simulink model "fourteen_bus_dynamic"  (Simulink 7.8)
settings: Solver=ode23t  StartTime=0.0  StopTime=5  FixedStep=0.2  RelTol=1e-4  AbsTol=1e-6
undefined symbols (not defined in the file or in its folder): D1, Delta
libraries: powerlib x56
settings Model: Creator=Bharath  LastModifiedBy=Bharath
settings SolverCC: MaxConsecutiveMinStep=auto  ZeroCrossControl=DisableAll
settings DataIOCC: LimitDataPoints=off  MaxDataPoints=500000
settings DebuggingCC: SolverPrmCheckMsg=none  UnconnectedOutputMsg=none

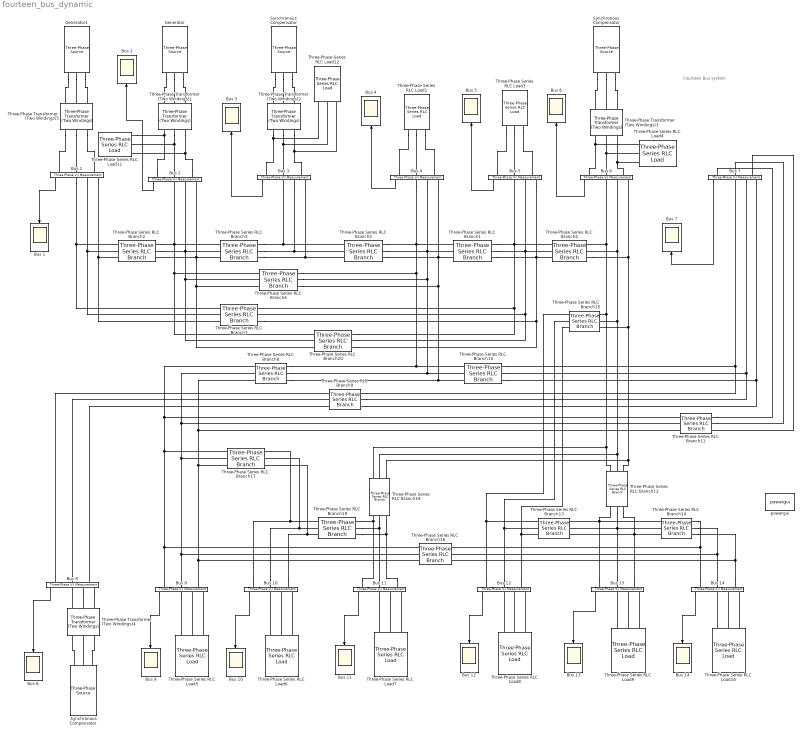
== system fourteen_bus_dynamic ==
  note: Fourteen Bus system
  " Generator" : powerlib/Electrical Sources/Three-Phase Source  Voltage=1.045  PhaseAngle=-30  Frequency=50  InternalConnection=Yg  SpecifyImpedance=on  Resistance=0.8929  Inductance=16.58e-3  ShortCircuitLevel=10  BaseVoltage=1  XRratio=1  BusType=PV  Pref=0.4  Qref=0  Qmin=-0.4  Qmax=0.5
  " Generator1" : powerlib/Electrical Sources/Three-Phase Source  Voltage=1.06  PhaseAngle=-30  Frequency=50  InternalConnection=Yg  SpecifyImpedance=on  Resistance=0.8929  Inductance=16.58e-3  ShortCircuitLevel=10  BaseVoltage=1  XRratio=1  BusType=PQ  Pref=2.324  Qref=-0.169  Qmin=0  Qmax=0
  Bus {1..14} (14 alike) : Scope
      Bus 1 settings: TimeRange=5  YMin=-1.75  YMax=1.75  SaveName=ScopeBus1
      Bus 10 settings: TimeRange=5  YMin=-1.5  YMax=1.5  SaveName=ScopeBus10
      Bus 11 settings: TickLabels=on  TimeRange=5  YMin=-1.25  YMax=1.25  SaveName=ScopeBus11
      Bus 12 settings: TimeRange=5  YMin=-1.25  YMax=1.25  SaveName=ScopeBus12
      Bus 13 settings: TimeRange=5  YMin=-1.25  YMax=1.25  SaveName=ScopeBus13
      Bus 14 settings: TimeRange=5  YMin=-1.25  YMax=1.25  SaveName=ScopeBus14
      Bus 2 settings: TimeRange=5  YMin=-1.75  YMax=1.75  SaveName=ScopeBus2
      Bus 3 settings: TimeRange=5  YMin=-1.75  YMax=1.75  SaveName=ScopeBus3
      Bus 4 settings: TimeRange=5  YMin=-1.25  YMax=1.25  SaveName=ScopeBus4
      Bus 5 settings: TimeRange=5  YMin=-1.75  YMax=2  SaveName=ScopeBus5
      Bus 6 settings: TimeRange=5  YMin=-1.75  YMax=1.75  SaveName=ScopeBus6
      Bus 7 settings: TimeRange=5  YMin=-1.25  YMax=1.25  SaveName=ScopeBus7
      Bus 8 settings: TimeRange=5  YMin=-1.1  YMax=1.1  SaveName=ScopeBus8
      Bus 9 settings: TimeRange=5  YMin=-1  YMax=0.9  SaveName=ScopeBus9
  "Bus 1 " : powerlib/Measurements/Three-Phase V-I Measurement  VoltageMeasurement=phase-to-ground  SetLabelV=off  LabelV=Vabc  Vpu=on  VpuLL=off  CurrentMeasurement=yes  SetLabelI=off  LabelI=Iabc  Ipu=on  Pbase=100e6  Vbase=0.95  OutputType=Complex  PhasorSimulation=off  PSBequivalent=0
  "Bus 10 " : powerlib/Measurements/Three-Phase V-I Measurement  VoltageMeasurement=phase-to-ground  SetLabelV=off  LabelV=Vabc  Vpu=on  VpuLL=off  CurrentMeasurement=yes  SetLabelI=off  LabelI=Iabc  Ipu=on  Pbase=100e6  Vbase=0.94  OutputType=Complex  PhasorSimulation=off  PSBequivalent=0
  "Bus 11 " : powerlib/Measurements/Three-Phase V-I Measurement  VoltageMeasurement=phase-to-ground  SetLabelV=off  LabelV=Vabc  Vpu=on  VpuLL=off  CurrentMeasurement=yes  SetLabelI=off  LabelI=Iabc  Ipu=on  Pbase=100e6  Vbase=0.95  OutputType=Complex  PhasorSimulation=off  PSBequivalent=0
  "Bus 12 " : powerlib/Measurements/Three-Phase V-I Measurement  VoltageMeasurement=phase-to-ground  SetLabelV=off  LabelV=Vabc  Vpu=on  VpuLL=off  CurrentMeasurement=yes  SetLabelI=off  LabelI=Iabc  Ipu=on  Pbase=100e6  Vbase=0.95  OutputType=Complex  PhasorSimulation=off  PSBequivalent=0
  "Bus 13 " : powerlib/Measurements/Three-Phase V-I Measurement  VoltageMeasurement=phase-to-ground  SetLabelV=off  LabelV=Vabc  Vpu=on  VpuLL=off  CurrentMeasurement=yes  SetLabelI=off  LabelI=Iabc  Ipu=on  Pbase=100e6  Vbase=0.95  OutputType=Complex  PhasorSimulation=off  PSBequivalent=0
  "Bus 14 " : powerlib/Measurements/Three-Phase V-I Measurement  VoltageMeasurement=phase-to-ground  SetLabelV=off  LabelV=Vabc  Vpu=on  VpuLL=off  CurrentMeasurement=yes  SetLabelI=off  LabelI=Iabc  Ipu=on  Pbase=100e6  Vbase=0.92  OutputType=Complex  PhasorSimulation=off  PSBequivalent=0
  "Bus 2 " : powerlib/Measurements/Three-Phase V-I Measurement  VoltageMeasurement=phase-to-ground  SetLabelV=off  LabelV=Vabc  Vpu=on  VpuLL=off  CurrentMeasurement=yes  SetLabelI=off  LabelI=Iabc  Ipu=on  Pbase=100e6  Vbase=0.95  OutputType=Complex  PhasorSimulation=off  PSBequivalent=0
  "Bus 3 " : powerlib/Measurements/Three-Phase V-I Measurement  VoltageMeasurement=phase-to-ground  SetLabelV=off  LabelV=Vabc  Vpu=on  VpuLL=off  CurrentMeasurement=yes  SetLabelI=off  LabelI=Iabc  Ipu=on  Pbase=100e6  Vbase=0.95  OutputType=Complex  PhasorSimulation=off  PSBequivalent=0
  "Bus 4 " : powerlib/Measurements/Three-Phase V-I Measurement  VoltageMeasurement=phase-to-ground  SetLabelV=off  LabelV=Vabc  Vpu=on  VpuLL=off  CurrentMeasurement=yes  SetLabelI=off  LabelI=Iabc  Ipu=on  Pbase=100e6  Vbase=0.95  OutputType=Complex  PhasorSimulation=off  PSBequivalent=0
  "Bus 5 " : powerlib/Measurements/Three-Phase V-I Measurement  VoltageMeasurement=phase-to-ground  SetLabelV=off  LabelV=Vabc  Vpu=on  VpuLL=off  CurrentMeasurement=yes  SetLabelI=off  LabelI=Iabc  Ipu=on  Pbase=100e6  Vbase=0.95  OutputType=Complex  PhasorSimulation=off  PSBequivalent=0
  "Bus 6 " : powerlib/Measurements/Three-Phase V-I Measurement  VoltageMeasurement=phase-to-ground  SetLabelV=off  LabelV=Vabc  Vpu=on  VpuLL=off  CurrentMeasurement=yes  SetLabelI=off  LabelI=Iabc  Ipu=on  Pbase=100e6  Vbase=0.95  OutputType=Complex  PhasorSimulation=off  PSBequivalent=0
  "Bus 7 " : powerlib/Measurements/Three-Phase V-I Measurement  VoltageMeasurement=phase-to-ground  SetLabelV=off  LabelV=Vabc  Vpu=on  VpuLL=off  CurrentMeasurement=yes  SetLabelI=off  LabelI=Iabc  Ipu=off  Pbase=100e6  Vbase=0.95  OutputType=Complex  PhasorSimulation=off  PSBequivalent=0
  "Bus 8 " : powerlib/Measurements/Three-Phase V-I Measurement  VoltageMeasurement=phase-to-ground  SetLabelV=off  LabelV=Vabc  Vpu=on  VpuLL=off  CurrentMeasurement=yes  SetLabelI=off  LabelI=Iabc  Ipu=on  Pbase=100e6  Vbase=1  OutputType=Complex  PhasorSimulation=off  PSBequivalent=0
  "Bus 9 " : powerlib/Measurements/Three-Phase V-I Measurement  VoltageMeasurement=phase-to-ground  SetLabelV=off  LabelV=Vabc  Vpu=on  VpuLL=off  CurrentMeasurement=yes  SetLabelI=off  LabelI=Iabc  Ipu=on  Pbase=100e6  Vbase=0.94  OutputType=Complex  PhasorSimulation=off  PSBequivalent=0
  Synchronous Compensator : powerlib/Electrical Sources/Three-Phase Source  Voltage=1.09  PhaseAngle=-30  Frequency=50  InternalConnection=Yg  SpecifyImpedance=on  Resistance=0.8929  Inductance=16.58e-3  ShortCircuitLevel=10  BaseVoltage=1  XRratio=1  BusType=PV  Pref=0  Qref=0  Qmin=-0.06  Qmax=0.24
  Synchronous  Compensator : powerlib/Electrical Sources/Three-Phase Source  Voltage=1.01  PhaseAngle=-30  Frequency=50  InternalConnection=Yg  SpecifyImpedance=on  Resistance=0.8929  Inductance=16.58e-3  ShortCircuitLevel=10  BaseVoltage=1  XRratio=1  BusType=PV  Pref=0  Qref=23.4e6  Qmin=0  Qmax=0.4
  "Synchronous  Compensator " : powerlib/Electrical Sources/Three-Phase Source  Voltage=1.07  PhaseAngle=-30  Frequency=50  InternalConnection=Yg  SpecifyImpedance=on  Resistance=0.8929  Inductance=16.58e-3  ShortCircuitLevel=10  BaseVoltage=1  XRratio=1  BusType=PV  Pref=0  Qref=23.4e6  Qmin=-0.06  Qmax=0.24
  Three-Phase Series RLC Branch1 : powerlib/Elements/Three-Phase Series RLC Branch  LConnTagsString=A|B|C  RConnTagsString=A|B|C  BranchType=RLC  Resistance=0.01335  Inductance=0.04211/(2*pi*50)  Capacitance=1/0.0128/(2*pi*50)  Measurements=None
  Three-Phase Series RLC Branch10 : powerlib/Elements/Three-Phase Series RLC Branch  LConnTagsString=A|B|C  RConnTagsString=A|B|C  BranchType=L  Resistance=1  Inductance=0.20912/(2*pi*50)  Capacitance=1e-6  Measurements=None
  Three-Phase Series RLC Branch11 : powerlib/Elements/Three-Phase Series RLC Branch  LConnTagsString=A|B|C  RConnTagsString=A|B|C  BranchType=L  Resistance=1  Inductance=0.11001/(2*pi*50)  Capacitance=1e-6  Measurements=None
  Three-Phase Series RLC Branch12 : powerlib/Elements/Three-Phase Series RLC Branch  LConnTagsString=A|B|C  RConnTagsString=A|B|C  BranchType=RL  Resistance=0.06615  Inductance=0.13027/(2*pi*50)  Capacitance=1e-6  Measurements=None
  Three-Phase Series RLC Branch13 : powerlib/Elements/Three-Phase Series RLC Branch  LConnTagsString=A|B|C  RConnTagsString=A|B|C  BranchType=RL  Resistance=0.22092  Inductance=0.19988/(2*pi*50)  Capacitance=1e-6  Measurements=None
  Three-Phase Series RLC Branch14 : powerlib/Elements/Three-Phase Series RLC Branch  LConnTagsString=A|B|C  RConnTagsString=A|B|C  BranchType=RL  Resistance=0.17093  Inductance=0.34802/(2*pi*50)  Capacitance=1e-6  Measurements=None
  Three-Phase Series RLC Branch15 : powerlib/Elements/Three-Phase Series RLC Branch  LConnTagsString=A|B|C  RConnTagsString=A|B|C  BranchType=RL  Resistance=0.12291  Inductance=0.25581/(2*pi*50)  Capacitance=1e-6  Measurements=None
  Three-Phase Series RLC Branch16 : powerlib/Elements/Three-Phase Series RLC Branch  LConnTagsString=A|B|C  RConnTagsString=A|B|C  BranchType=RL  Resistance=0.12711  Inductance=0.27038/(2*pi*50)  Capacitance=1e-6  Measurements=None
  Three-Phase Series RLC Branch17 : powerlib/Elements/Three-Phase Series RLC Branch  LConnTagsString=A|B|C  RConnTagsString=A|B|C  BranchType=RL  Resistance=0.03181  Inductance=0.08450/(2*pi*50)  Capacitance=1e-6  Measurements=None
  Three-Phase Series RLC Branch18 : powerlib/Elements/Three-Phase Series RLC Branch  LConnTagsString=A|B|C  RConnTagsString=A|B|C  BranchType=RL  Resistance=0.09498  Inductance=0.1989/(2*pi*50)  Capacitance=1e-6  Measurements=None
  Three-Phase Series RLC Branch19 : powerlib/Elements/Three-Phase Series RLC Branch  LConnTagsString=A|B|C  RConnTagsString=A|B|C  BranchType=RL  Resistance=0.08205  Inductance=0.19207/(2*pi*50)  Capacitance=1e-6  Measurements=None
  Three-Phase Series RLC Branch2 : powerlib/Elements/Three-Phase Series RLC Branch  LConnTagsString=A|B|C  RConnTagsString=A|B|C  BranchType=RLC  Resistance=0.01938  Inductance=0.05917/(2*pi*50)  Capacitance=1/0.0528/(2*pi*50)  Measurements=None
  Three-Phase Series RLC Branch20 : powerlib/Elements/Three-Phase Series RLC Branch  LConnTagsString=A|B|C  RConnTagsString=A|B|C  BranchType=RLC  Resistance=0.05695  Inductance=0.17388/(2*pi*50)  Capacitance=1/0.0340/(2*pi*50)  Measurements=None
  Three-Phase Series RLC Branch3 : powerlib/Elements/Three-Phase Series RLC Branch  LConnTagsString=A|B|C  RConnTagsString=A|B|C  BranchType=RLC  Resistance=0.04699  Inductance=0.19797/(2*pi*50)  Capacitance=1/0.0438/(2*pi*50)  Measurements=None
  Three-Phase Series RLC Branch4 : powerlib/Elements/Three-Phase Series RLC Branch  LConnTagsString=A|B|C  RConnTagsString=A|B|C  BranchType=L  Resistance=1  Inductance=0.25202/(2*pi*50)  Capacitance=1e-6  Measurements=None
  Three-Phase Series RLC Branch5 : powerlib/Elements/Three-Phase Series RLC Branch  LConnTagsString=A|B|C  RConnTagsString=A|B|C  BranchType=RLC  Resistance=0.06701  Inductance=0.17103/(2*pi*50)  Capacitance=1/0.0346/(2*pi*50)  Measurements=None
  Three-Phase Series RLC Branch6 : powerlib/Elements/Three-Phase Series RLC Branch  LConnTagsString=A|B|C  RConnTagsString=A|B|C  BranchType=RLC  Resistance=0.05811  Inductance=0.17632/(2*pi*50)  Capacitance=1/0.0374/(2*pi*50)  Measurements=None
  Three-Phase Series RLC Branch7 : powerlib/Elements/Three-Phase Series RLC Branch  LConnTagsString=A|B|C  RConnTagsString=A|B|C  BranchType=RLC  Resistance=0.05403  Inductance=0.22304/(2*pi*50)  Capacitance=1/0.0492/(2*pi*50)  Measurements=None
  Three-Phase Series RLC Branch8 : powerlib/Elements/Three-Phase Series RLC Branch  LConnTagsString=A|B|C  RConnTagsString=A|B|C  BranchType=L  Resistance=1  Inductance=0.55618/(2*pi*50)  Capacitance=1e-6  Measurements=None
  Three-Phase Series RLC Branch9 : powerlib/Elements/Three-Phase Series RLC Branch  LConnTagsString=A|B|C  RConnTagsString=A|B|C  BranchType=L  Resistance=1  Inductance=0.17615/(2*pi*50)  Capacitance=1e-6  Measurements=None
  Three-Phase Series RLC Load1 : powerlib/Elements/Three-Phase Series RLC Load  LConnTagsString=A|B|C  Configuration=Y (grounded)  NominalVoltage=1  NominalFrequency=50  ActivePower=0.478  InductivePower=0  CapacitivePower=0.039  Measurements=None  LoadType=constant PQ
  Three-Phase Series RLC Load10 : powerlib/Elements/Three-Phase Series RLC Load  LConnTagsString=A|B|C  Configuration=Y (grounded)  NominalVoltage=1  NominalFrequency=50  ActivePower=0.149  InductivePower=0.050  CapacitivePower=0  Measurements=None  LoadType=constant Z
  Three-Phase Series RLC Load11 : powerlib/Elements/Three-Phase Series RLC Load  LConnTagsString=A|B|C  Configuration=Y (grounded)  NominalVoltage=1  NominalFrequency=50  ActivePower=0.217  InductivePower=0.127  CapacitivePower=0  Measurements=None  LoadType=constant PQ
  Three-Phase Series RLC Load12 : powerlib/Elements/Three-Phase Series RLC Load  LConnTagsString=A|B|C  Configuration=Y (grounded)  NominalVoltage=1  NominalFrequency=50  ActivePower=0.942  InductivePower=0.191  CapacitivePower=0  Measurements=None  LoadType=constant PQ
  Three-Phase Series RLC Load3 : powerlib/Elements/Three-Phase Series RLC Load  LConnTagsString=A|B|C  Configuration=Y (grounded)  NominalVoltage=1  NominalFrequency=50  ActivePower=0.076  InductivePower=0.016  CapacitivePower=0  Measurements=None  LoadType=constant PQ
  Three-Phase Series RLC Load4 : powerlib/Elements/Three-Phase Series RLC Load  LConnTagsString=A|B|C  Configuration=Y (grounded)  NominalVoltage=1  NominalFrequency=50  ActivePower=0.112  InductivePower=0.075  CapacitivePower=0  Measurements=None  LoadType=constant PQ
  Three-Phase Series RLC Load5 : powerlib/Elements/Three-Phase Series RLC Load  LConnTagsString=A|B|C  Configuration=Y (grounded)  NominalVoltage=1  NominalFrequency=50  ActivePower=0.295  InductivePower=0.166  CapacitivePower=0  Measurements=None  LoadType=constant PQ
  Three-Phase Series RLC Load6 : powerlib/Elements/Three-Phase Series RLC Load  LConnTagsString=A|B|C  Configuration=Y (grounded)  NominalVoltage=1  NominalFrequency=50  ActivePower=0.09  InductivePower=0.058  CapacitivePower=0  Measurements=None  LoadType=constant PQ
  Three-Phase Series RLC Load7 : powerlib/Elements/Three-Phase Series RLC Load  LConnTagsString=A|B|C  Configuration=Y (grounded)  NominalVoltage=1  NominalFrequency=50  ActivePower=0.035  InductivePower=0.018  CapacitivePower=0  Measurements=None  LoadType=constant PQ
  Three-Phase Series RLC Load8 : powerlib/Elements/Three-Phase Series RLC Load  LConnTagsString=A|B|C  Configuration=Y (grounded)  NominalVoltage=1  NominalFrequency=50  ActivePower=0.061  InductivePower=0.016  CapacitivePower=0  Measurements=None  LoadType=constant PQ
  Three-Phase Series RLC Load9 : powerlib/Elements/Three-Phase Series RLC Load  LConnTagsString=A|B|C  Configuration=Y (grounded)  NominalVoltage=1  NominalFrequency=50  ActivePower=0.135  InductivePower=0.058  CapacitivePower=0  Measurements=None  LoadType=constant PQ
  Three-Phase Transformer (Two Windings)1 : powerlib/Elements/Three-Phase Transformer (Two Windings)  Winding1Connection=Delta (D1)  UNITS=pu  NominalPower=[ 1 , 50 ]  Winding1=[ 1.045 , 0.002 , 0.08 ]  Winding2Connection=Yg  Winding2=[ 1.045 , 0.002 , 0.08 ]  SetSaturation=off  Rm=500  Lm=500  Saturation=[ 0,0 ; 0.0024,1.2 ; 1.0,1.52 ]  Hysteresis=off  DataFile='hysteresis'  SetInitialFlux=off  InitialFluxes=[ 0.8 , -0.8 , 0.7 ]  Measurements=None  MoreParameters=off  BreakLoop=off  DataType=off  TransfoNumber=1
  Three-Phase Transformer (Two Windings)2 : powerlib/Elements/Three-Phase Transformer (Two Windings)  Winding1Connection=Delta (D1)  UNITS=pu  NominalPower=[ 1 , 50 ]  Winding1=[ 1.01 , 0.002 , 0.08 ]  Winding2Connection=Yg  Winding2=[ 1.01 , 0.002 , 0.08 ]  SetSaturation=off  Rm=500  Lm=500  Saturation=[ 0,0 ; 0.0024,1.2 ; 1.0,1.52 ]  Hysteresis=off  DataFile='hysteresis'  SetInitialFlux=off  InitialFluxes=[ 0.8 , -0.8 , 0.7 ]  Measurements=None  MoreParameters=off  BreakLoop=off  DataType=off  TransfoNumber=1
  Three-Phase Transformer (Two Windings)3 : powerlib/Elements/Three-Phase Transformer (Two Windings)  Winding1Connection=Delta (D1)  UNITS=pu  NominalPower=[ 1 , 50 ]  Winding1=[ 1.07 , 0.002 , 0.08 ]  Winding2Connection=Yg  Winding2=[ 1.07 , 0.002 , 0.08 ]  SetSaturation=off  Rm=500  Lm=500  Saturation=[ 0,0 ; 0.0024,1.2 ; 1.0,1.52 ]  Hysteresis=off  DataFile='hysteresis'  SetInitialFlux=off  InitialFluxes=[ 0.8 , -0.8 , 0.7 ]  Measurements=None  MoreParameters=off  BreakLoop=off  DataType=off  TransfoNumber=1
  Three-Phase Transformer (Two Windings)4 : powerlib/Elements/Three-Phase Transformer (Two Windings)  Winding1Connection=Yg  UNITS=pu  NominalPower=[ 1 , 50 ]  Winding1=[ 1.09 , 0.002 , 0.08]  Winding2Connection=Delta (D1)  Winding2=[1.09 , 0.002 , 0.08]  SetSaturation=off  Rm=500  Lm=500  Saturation=[0 0;0.0023999 1.2;1 1.52]  Hysteresis=off  DataFile='hysteresis'  SetInitialFlux=off  InitialFluxes=[0.80002 -0.80002 0.69999]  Measurements=None  MoreParameters=off  BreakLoop=off  DataType=off  TransfoNumber=1
  Three-Phase Transformer (Two Windings)5 : powerlib/Elements/Three-Phase Transformer (Two Windings)  Winding1Connection=Delta (D1)  UNITS=pu  NominalPower=[ 1 , 50 ]  Winding1=[ 1.06 , 0.002 , 0.08 ]  Winding2Connection=Yg  Winding2=[ 1.06 , 0.002 , 0.08 ]  SetSaturation=off  Rm=500  Lm=500  Saturation=[ 0,0 ; 0.0024,1.2 ; 1.0,1.52 ]  Hysteresis=off  DataFile='hysteresis'  SetInitialFlux=off  InitialFluxes=[ 0.8 , -0.8 , 0.7 ]  Measurements=None  MoreParameters=off  BreakLoop=off  DataType=off  TransfoNumber=1
  powergui : powerlib/powergui  Priority=1  SimulationMode=Continuous  SolverType=Tustin  SampleTime=50e-6  frequency=60  SPID=off  DisableSnubberDevices=off  DisableRonSwitches=off  DisableVfSwitches=off  SwTol=0  Interpol=off  DisplayEquations=off  FunctionMessages=off  frequencyindice=0  Pbase=100e6  ErrMax=1e-4  Iterations=50  UnitsV=kV  UnitsW=MW  echomessages=off  HookPort=off  EnableUseOfTLC=off  x0status=blocks  RestoreLinks=warning  ResistiveCurrentMeasurement=off  Ylog=off  Xlog=on  ShowGrid=off  save=off  variable=ZData  ZoomFFT=off  StartTime=0.0  cycles=1  DisplayStyle=1  FreqAxis=off  MaxFrequency=1000  frequencyindicesteady=1  display=off  methode=off
  wires:
  "Bus 11 "/1 -> Bus 11/1
  "Bus 10 "/1 -> Bus 10/1
  "Bus 9 "/1 -> Bus 9/1
  "Bus 8 "/1 -> Bus 8/1
  "Bus 7 "/1 -> Bus 7/1
  "Bus 4 "/1 -> Bus 4/1
  "Bus 2 "/1 -> Bus 2/1
  "Bus 14 "/1 -> Bus 14/1
  "Bus 13 "/1 -> Bus 13/1
  "Bus 12 "/1 -> Bus 12/1
  "Bus 5 "/1 -> Bus 5/1
  "Bus 1 "/1 -> Bus 1/1
  "Bus 3 "/1 -> Bus 3/1
  "Bus 6 "/1 -> Bus 6/1
  connections:
  "Bus 9 "/LConn3 -- Three-Phase Series RLC Branch16/RConn3 -- Three-Phase Series RLC Branch17/RConn3 -- Three-Phase Series RLC Branch11/RConn3 -- Three-Phase Series RLC Branch8/LConn3
  "Bus 9 "/LConn2 -- Three-Phase Series RLC Branch16/RConn2 -- Three-Phase Series RLC Branch17/RConn2 -- Three-Phase Series RLC Branch11/RConn2 -- Three-Phase Series RLC Branch8/LConn2
  "Bus 9 "/LConn1 -- Three-Phase Series RLC Branch16/RConn1 -- Three-Phase Series RLC Branch17/RConn1 -- Three-Phase Series RLC Branch11/RConn1 -- Three-Phase Series RLC Branch8/LConn1
  "Bus 7 "/RConn3 -- Three-Phase Series RLC Branch10/RConn3 -- Three-Phase Series RLC Branch9/RConn3
  "Bus 7 "/RConn2 -- Three-Phase Series RLC Branch10/RConn2 -- Three-Phase Series RLC Branch9/RConn2
  "Bus 7 "/RConn1 -- Three-Phase Series RLC Branch10/RConn1 -- Three-Phase Series RLC Branch9/RConn1
  "Bus 6 "/RConn3 -- Three-Phase Series RLC Branch4/RConn3 -- Three-Phase Series RLC Branch12/LConn3 -- Three-Phase Series RLC Branch18/LConn3 -- Three-Phase Series RLC Branch15/LConn3
  "Bus 6 "/RConn2 -- Three-Phase Series RLC Branch15/LConn2 -- Three-Phase Series RLC Branch18/LConn2 -- Three-Phase Series RLC Branch12/LConn2 -- Three-Phase Series RLC Branch4/RConn2
  "Bus 6 "/RConn1 -- Three-Phase Series RLC Branch12/LConn1 -- Three-Phase Series RLC Branch18/LConn1 -- Three-Phase Series RLC Branch15/LConn1 -- Three-Phase Series RLC Branch4/RConn1
  "Bus 5 "/RConn3 -- Three-Phase Series RLC Branch1/RConn3 -- Three-Phase Series RLC Branch20/RConn3 -- Three-Phase Series RLC Branch7/RConn3 -- Three-Phase Series RLC Branch4/LConn3
  "Bus 5 "/RConn2 -- Three-Phase Series RLC Branch1/RConn2 -- Three-Phase Series RLC Branch20/RConn2 -- Three-Phase Series RLC Branch7/RConn2 -- Three-Phase Series RLC Branch4/LConn2
  "Bus 5 "/RConn1 -- Three-Phase Series RLC Branch1/RConn1 -- Three-Phase Series RLC Branch20/RConn1 -- Three-Phase Series RLC Branch7/RConn1 -- Three-Phase Series RLC Branch4/LConn1
  "Bus 3 "/RConn2 -- Three-Phase Series RLC Branch5/LConn2 -- Three-Phase Series RLC Branch3/RConn2
  "Bus 3 "/RConn1 -- Three-Phase Series RLC Branch5/LConn1 -- Three-Phase Series RLC Branch3/RConn1
  "Bus 2 "/RConn3 -- Three-Phase Series RLC Branch20/LConn3 -- Three-Phase Series RLC Branch6/LConn3 -- Three-Phase Series RLC Branch3/LConn3 -- Three-Phase Series RLC Branch2/RConn3
  "Bus 2 "/RConn2 -- Three-Phase Series RLC Branch20/LConn2 -- Three-Phase Series RLC Branch6/LConn2 -- Three-Phase Series RLC Branch2/RConn2 -- Three-Phase Series RLC Branch3/LConn2
  "Bus 2 "/RConn1 -- Three-Phase Series RLC Branch20/LConn1 -- Three-Phase Series RLC Branch6/LConn1 -- Three-Phase Series RLC Branch2/RConn1 -- Three-Phase Series RLC Branch3/LConn1
  "Bus 2 "/LConn2 -- Three-Phase Series RLC Load11/LConn2 -- Three-Phase Transformer (Two Windings)1/RConn2
  "Bus 2 "/LConn1 -- Three-Phase Series RLC Load11/LConn1 -- Three-Phase Transformer (Two Windings)1/RConn1
  "Bus 14 "/LConn3 -- Three-Phase Series RLC Branch16/LConn3 -- Three-Phase Series RLC Branch14/LConn3
  "Bus 14 "/LConn2 -- Three-Phase Series RLC Branch16/LConn2 -- Three-Phase Series RLC Branch14/LConn2
  "Bus 14 "/LConn1 -- Three-Phase Series RLC Branch16/LConn1 -- Three-Phase Series RLC Branch14/LConn1
  "Bus 13 "/LConn3 -- Three-Phase Series RLC Branch14/RConn3 -- Three-Phase Series RLC Branch13/LConn3 -- Three-Phase Series RLC Branch12/RConn3
  "Bus 13 "/LConn2 -- Three-Phase Series RLC Branch14/RConn2 -- Three-Phase Series RLC Branch12/RConn2 -- Three-Phase Series RLC Branch13/LConn2
  "Bus 13 "/LConn1 -- Three-Phase Series RLC Branch14/RConn1 -- Three-Phase Series RLC Branch12/RConn1 -- Three-Phase Series RLC Branch13/LConn1
  "Bus 12 "/LConn3 -- Three-Phase Series RLC Branch13/RConn3 -- Three-Phase Series RLC Branch15/RConn3
  "Bus 12 "/LConn2 -- Three-Phase Series RLC Branch13/RConn2 -- Three-Phase Series RLC Branch15/RConn2
  "Bus 12 "/LConn1 -- Three-Phase Series RLC Branch13/RConn1 -- Three-Phase Series RLC Branch15/RConn1
  "Bus 11 "/LConn3 -- Three-Phase Series RLC Branch19/RConn3 -- Three-Phase Series RLC Branch18/RConn3
  "Bus 11 "/LConn2 -- Three-Phase Series RLC Branch19/RConn2 -- Three-Phase Series RLC Branch18/RConn2
  "Bus 11 "/LConn1 -- Three-Phase Series RLC Branch19/RConn1 -- Three-Phase Series RLC Branch18/RConn1
  "Bus 10 "/LConn3 -- Three-Phase Series RLC Branch17/LConn3 -- Three-Phase Series RLC Branch19/LConn3
  "Bus 10 "/LConn2 -- Three-Phase Series RLC Branch17/LConn2 -- Three-Phase Series RLC Branch19/LConn2
  "Bus 10 "/LConn1 -- Three-Phase Series RLC Branch17/LConn1 -- Three-Phase Series RLC Branch19/LConn1
  "Bus 1 "/RConn3 -- Three-Phase Series RLC Branch2/LConn3 -- Three-Phase Series RLC Branch7/LConn3
  "Bus 1 "/RConn2 -- Three-Phase Series RLC Branch2/LConn2 -- Three-Phase Series RLC Branch7/LConn2
  "Bus 1 "/RConn1 -- Three-Phase Series RLC Branch2/LConn1 -- Three-Phase Series RLC Branch7/LConn1
  Three-Phase Series RLC Load1/LConn3 -- "Bus 4 "/LConn3
  "Bus 8 "/RConn3 -- Three-Phase Transformer (Two Windings)4/LConn3
  "Bus 8 "/RConn2 -- Three-Phase Transformer (Two Windings)4/LConn2
  Three-Phase Transformer (Two Windings)4/LConn1 -- "Bus 8 "/RConn1
  Three-Phase Series RLC Load5/LConn2 -- "Bus 9 "/RConn2
  "Bus 9 "/RConn1 -- Three-Phase Series RLC Load5/LConn1
  Three-Phase Series RLC Load5/LConn3 -- "Bus 9 "/RConn3
  " Generator"/RConn2 -- Three-Phase Transformer (Two Windings)1/LConn2
  Three-Phase Series RLC Load1/LConn2 -- "Bus 4 "/LConn2
  Three-Phase Series RLC Load3/LConn1 -- "Bus 5 "/LConn1
  Three-Phase Series RLC Load3/LConn3 -- "Bus 5 "/LConn3
  "Bus 7 "/LConn3 -- Three-Phase Series RLC Branch11/LConn3
  Three-Phase Series RLC Load3/LConn2 -- "Bus 5 "/LConn2
  Three-Phase Series RLC Load10/LConn3 -- "Bus 14 "/RConn3
  Three-Phase Series RLC Load10/LConn2 -- "Bus 14 "/RConn2
  Three-Phase Series RLC Load10/LConn1 -- "Bus 14 "/RConn1
  Three-Phase Series RLC Load9/LConn3 -- "Bus 13 "/RConn3
  Three-Phase Series RLC Load9/LConn2 -- "Bus 13 "/RConn2
  Three-Phase Series RLC Load9/LConn1 -- "Bus 13 "/RConn1
  Three-Phase Series RLC Load8/LConn3 -- "Bus 12 "/RConn3
  Three-Phase Series RLC Load8/LConn2 -- "Bus 12 "/RConn2
  Three-Phase Series RLC Load8/LConn1 -- "Bus 12 "/RConn1
  Three-Phase Series RLC Load7/LConn3 -- "Bus 11 "/RConn3
  "Bus 11 "/RConn2 -- Three-Phase Series RLC Load7/LConn2
  "Bus 11 "/RConn1 -- Three-Phase Series RLC Load7/LConn1
  Three-Phase Series RLC Load6/LConn3 -- "Bus 10 "/RConn3
  Three-Phase Series RLC Load6/LConn2 -- "Bus 10 "/RConn2
  Three-Phase Series RLC Load6/LConn1 -- "Bus 10 "/RConn1
  "Bus 2 "/LConn3 -- Three-Phase Series RLC Load11/LConn3 -- Three-Phase Transformer (Two Windings)1/RConn3
  Three-Phase Series RLC Branch9/LConn1 -- "Bus 8 "/LConn1
  Three-Phase Series RLC Branch9/LConn2 -- "Bus 8 "/LConn2
  Three-Phase Series RLC Branch9/LConn3 -- "Bus 8 "/LConn3
  Three-Phase Series RLC Load1/LConn1 -- "Bus 4 "/LConn1
  Three-Phase Series RLC Branch11/LConn2 -- "Bus 7 "/LConn2
  Three-Phase Series RLC Branch11/LConn1 -- "Bus 7 "/LConn1
  Three-Phase Transformer (Two Windings)5/RConn2 -- "Bus 1 "/LConn2
  Three-Phase Transformer (Two Windings)5/RConn1 -- "Bus 1 "/LConn1
  " Generator1"/RConn2 -- Three-Phase Transformer (Two Windings)5/LConn2
  Three-Phase Transformer (Two Windings)5/RConn3 -- "Bus 1 "/LConn3
  Three-Phase Series RLC Load12/LConn2 -- Three-Phase Transformer (Two Windings)2/RConn2 -- "Bus 3 "/LConn2
  Three-Phase Series RLC Load12/LConn1 -- Three-Phase Transformer (Two Windings)2/RConn1 -- "Bus 3 "/LConn1
  Synchronous  Compensator/RConn2 -- Three-Phase Transformer (Two Windings)2/LConn2
  Three-Phase Series RLC Load12/LConn3 -- Three-Phase Transformer (Two Windings)2/RConn3 -- "Bus 3 "/LConn3
  "Bus 6 "/LConn2 -- Three-Phase Transformer (Two Windings)3/RConn2 -- Three-Phase Series RLC Load4/LConn2
  "Bus 6 "/LConn1 -- Three-Phase Transformer (Two Windings)3/RConn1 -- Three-Phase Series RLC Load4/LConn1
  Three-Phase Transformer (Two Windings)3/RConn3 -- "Bus 6 "/LConn3 -- Three-Phase Series RLC Load4/LConn3
  "Synchronous  Compensator "/RConn2 -- Three-Phase Transformer (Two Windings)3/LConn2
  "Bus 4 "/RConn3 -- Three-Phase Series RLC Branch1/LConn3 -- Three-Phase Series RLC Branch5/RConn3 -- Three-Phase Series RLC Branch6/RConn3 -- Three-Phase Series RLC Branch10/LConn3 -- Three-Phase Series RLC Branch8/RConn3
  "Bus 4 "/RConn2 -- Three-Phase Series RLC Branch1/LConn2 -- Three-Phase Series RLC Branch6/RConn2 -- Three-Phase Series RLC Branch10/LConn2 -- Three-Phase Series RLC Branch8/RConn2 -- Three-Phase Series RLC Branch5/RConn2
  "Bus 4 "/RConn1 -- Three-Phase Series RLC Branch1/LConn1 -- Three-Phase Series RLC Branch6/RConn1 -- Three-Phase Series RLC Branch10/LConn1 -- Three-Phase Series RLC Branch8/RConn1 -- Three-Phase Series RLC Branch5/RConn1
  Synchronous Compensator/RConn2 -- Three-Phase Transformer (Two Windings)4/RConn2
  Synchronous Compensator/RConn3 -- Three-Phase Transformer (Two Windings)4/RConn3
  Synchronous Compensator/RConn1 -- Three-Phase Transformer (Two Windings)4/RConn1
  "Synchronous  Compensator "/RConn1 -- Three-Phase Transformer (Two Windings)3/LConn1
  "Synchronous  Compensator "/RConn3 -- Three-Phase Transformer (Two Windings)3/LConn3
  " Generator1"/RConn3 -- Three-Phase Transformer (Two Windings)5/LConn3
  " Generator1"/RConn1 -- Three-Phase Transformer (Two Windings)5/LConn1
  Synchronous  Compensator/RConn3 -- Three-Phase Transformer (Two Windings)2/LConn3
  Synchronous  Compensator/RConn1 -- Three-Phase Transformer (Two Windings)2/LConn1
  " Generator"/RConn1 -- Three-Phase Transformer (Two Windings)1/LConn1
  " Generator"/RConn3 -- Three-Phase Transformer (Two Windings)1/LConn3
  "Bus 3 "/RConn3 -- Three-Phase Series RLC Branch5/LConn3 -- Three-Phase Series RLC Branch3/RConn3
